simulink model "Non_linear_bicycle_model"  (R2020a)
settings: Solver=VariableStepAuto  StartTime=0.0  StopTime=10.0  RelTol=1e-3
values from neighbouring files (symbols this model uses):
  c_alpha_f = 156000    [init.m]
  c_alpha_r = 193000    [init.m]
  delta_max = deg2rad(37.3)    [init.m]
  g = 9.81    [init.m]
  Iz = 2937    [init.m]
  lf = 1.04    [init.m]
  lr = 1.40    (= 1.4)    [init.m]
  mass = 1919    [init.m]
  psi0 = 0*pi/180    (= 0)    [init.m]
  psid0 = 0    [init.m]
  steering_constant = deg2rad(10)    [init.m]
  steering_input_switch = 3    [init.m]
  steering_omega = 0.25    [init.m]
  steering_rate = deg2rad(2)    [init.m]
  v_lat0 = 0    [init.m]
  v_lon0 = 5    [init.m]
  wff = 0.577    [init.m]
  wfr = 0.423    [init.m]
  x0 = 0    [init.m]
  y0 = 0    [init.m]
undefined symbols (not defined in the file or in its folder): B_f, B_r, C_f, C_r, coefficient_friction, D_f, D_r, E_f, E_r
libraries: simulink x2
settings Model: Creator=Sameed Quais  LastModifiedBy=Sameed Quais

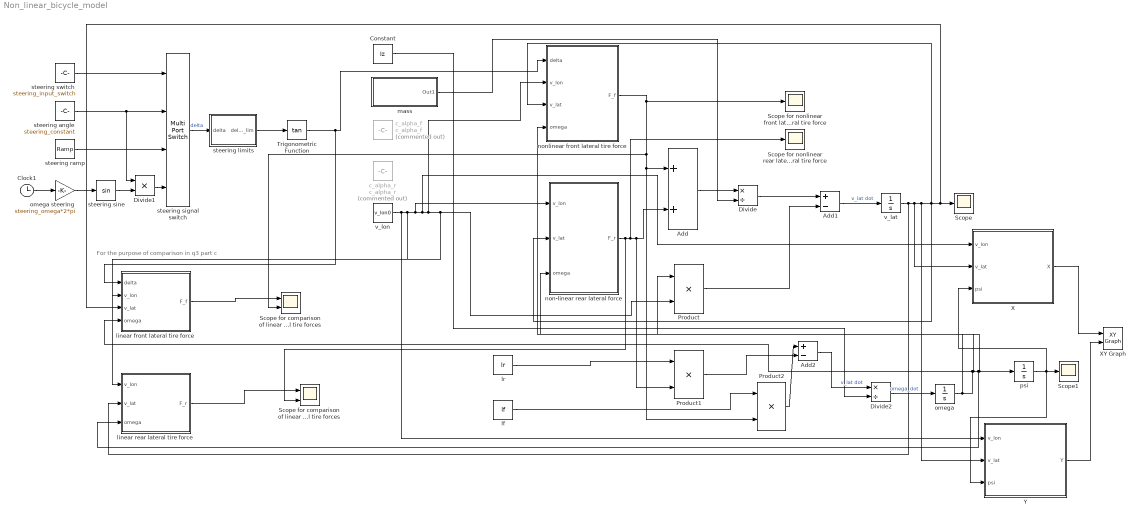
== system Non_linear_bicycle_model ==
  note: For the purpose of comparison in q3 part c
  Add : Sum
  Add1 : Sum  Inputs=+-
  Add2 : Sum  Inputs=+-
  Clock1 : Clock
  Constant : Constant  Value=Iz
  Divide : Product  Inputs=*/
  Divide1 : Product
  Divide2 : Product  Inputs=*/
  Product : Product
  Product1 : Product
  Product2 : Product
  Scope : Scope
  Scope for comparison of linear and non-linear front lateral tire forces : Scope  NumInputPorts=2
  Scope for comparison of linear and non-linear rear lateral tire forces : Scope  NumInputPorts=2
  Scope for nonlinear front lateral tire force : Scope
  Scope for nonlinear rear lateral tire force : Scope
  Scope1 : Scope
  Trigonometric Function : Trigonometry  Operator=tan
  X : Subsystem
  XY Graph : simulink/Sinks/XY Graph  xmin=-inf  xmax=inf  ymin=-inf  ymax=inf  st=-1
  Y : Subsystem
  c_alpha_f : Constant  Commented=on  Value=c_alpha_f
  c_alpha_r : Constant  Commented=on  Value=c_alpha_r
  lf : Constant  Value=lf
  linear front lateral tire force : Subsystem
  linear rear lateral tire force : Subsystem
  lr : Constant  Value=lr
  mass : Subsystem
  non-linear rear lateral force : Subsystem
  nonlinear front lateral tire force : Subsystem
  omega : Integrator  InitialCondition=psi0
  omega steering : Gain  Gain=steering_omega*2*pi
  psi : Integrator  InitialCondition=psid0
  steering angle : Constant  Value=steering_constant
  steering limits : Subsystem
  steering ramp : simulink/Sources/Ramp  slope=steering_rate  start=0  InitialOutput=0
  steering sine : Trigonometry
  steering switch : Constant  Value=steering_input_switch
  steering signal switch : MultiPortSwitch
  v_lat : Integrator  InitialCondition=v_lat0
  v_lon : Constant  Value=v_lon0
  wires:
  non-linear rear lateral force/1(F_r) -> Scope for nonlinear rear lateral tire force/1, Product1/2, Add/2, Scope for comparison of linear and non-linear rear lateral tire forces/2
  nonlinear front lateral tire force/1(F_f) -> Scope for comparison of linear and non-linear front lateral tire forces/2, Product2/2, Add/1, Scope for nonlinear front lateral tire force/1
  Add/1 -> Divide/1
  mass/1(Out1) -> Divide/2
  Divide/1 -> Add1/1
  v_lon/1 -> Y/1(v_lon), linear front lateral tire force/2(v_lon), non-linear rear lateral force/1(v_lon), X/1(v_lon), nonlinear front lateral tire force/2(v_lon), linear rear lateral tire force/1(v_lon), Product/2
  Product/1 -> Add1/2
  Add1/1 -> v_lat/1  "v_lat dot"
  lr/1 -> Product1/1
  lf/1 -> Product2/1
  Product2/1 -> Add2/1
  Product1/1 -> Add2/2
  Constant/1 -> Divide2/2
  Add2/1 -> Divide2/1  "v_lat dot"
  Divide2/1 -> omega/1  "omega_dot"
  v_lat/1 -> linear rear lateral tire force/2(v_lat), X/2(v_lat), Y/2(v_lat), non-linear rear lateral force/2(v_lat), nonlinear front lateral tire force/3(v_lat), linear front lateral tire force/3(v_lat), Scope/1
  omega/1 -> non-linear rear lateral force/3(omega), linear front lateral tire force/4(omega), Product/1, psi/1, nonlinear front lateral tire force/4(omega), linear rear lateral tire force/3(omega)
  steering limits/1(delta_lim) -> Trigonometric Function/1
  steering signal switch/1 -> steering limits/1(delta)  "delta"
  Clock1/1 -> omega steering/1
  steering angle/1 -> Divide1/1, steering signal switch/2
  Divide1/1 -> steering signal switch/4
  omega steering/1 -> steering sine/1
  steering switch/1 -> steering signal switch/1
  steering ramp/1 -> steering signal switch/3
  steering sine/1 -> Divide1/2
  Trigonometric Function/1 -> linear front lateral tire force/1(delta), nonlinear front lateral tire force/1(delta)
  psi/1 -> Y/3(psi), X/3(psi), Scope1/1
  X/1(X) -> XY Graph/1
  Y/1(Y) -> XY Graph/2
  linear front lateral tire force/1(F_f) -> Scope for comparison of linear and non-linear front lateral tire forces/1
  linear rear lateral tire force/1(F_r) -> Scope for comparison of linear and non-linear rear lateral tire forces/1

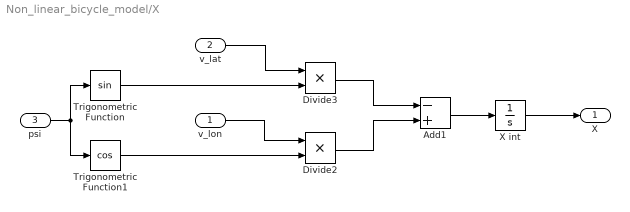
== system Non_linear_bicycle_model/X ==
  v_lon : Inport
  v_lat : Inport  Port=2
  psi : Inport  Port=3
  Add1 : Sum  Inputs=-+
  Divide2 : Product
  Divide3 : Product
  Trigonometric Function : Trigonometry
  Trigonometric Function1 : Trigonometry  Operator=cos
  X int : Integrator  InitialCondition=x0
  X : Outport  VectorParamsAs1DForOutWhenUnconnected=off
  wires:
  Add1/1 -> X int/1
  v_lon/1 -> Divide2/1
  Divide2/1 -> Add1/2
  v_lat/1 -> Divide3/1
  psi/1 -> Trigonometric Function/1, Trigonometric Function1/1
  Trigonometric Function1/1 -> Divide2/2
  Trigonometric Function/1 -> Divide3/2
  Divide3/1 -> Add1/1
  X int/1 -> X/1

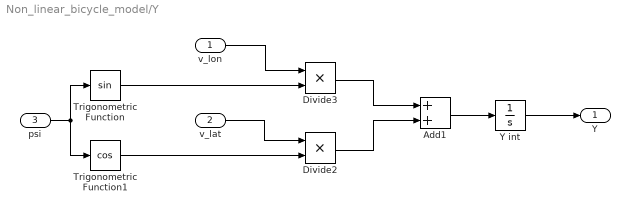
== system Non_linear_bicycle_model/Y ==
  v_lon : Inport
  v_lat : Inport  Port=2
  psi : Inport  Port=3
  Add1 : Sum
  Divide2 : Product
  Divide3 : Product
  Trigonometric Function : Trigonometry
  Trigonometric Function1 : Trigonometry  Operator=cos
  Y int : Integrator  InitialCondition=y0
  Y : Outport  VectorParamsAs1DForOutWhenUnconnected=off
  wires:
  Add1/1 -> Y int/1
  v_lat/1 -> Divide2/1
  Divide2/1 -> Add1/2
  v_lon/1 -> Divide3/1
  psi/1 -> Trigonometric Function/1, Trigonometric Function1/1
  Trigonometric Function1/1 -> Divide2/2
  Trigonometric Function/1 -> Divide3/2
  Divide3/1 -> Add1/1
  Y int/1 -> Y/1

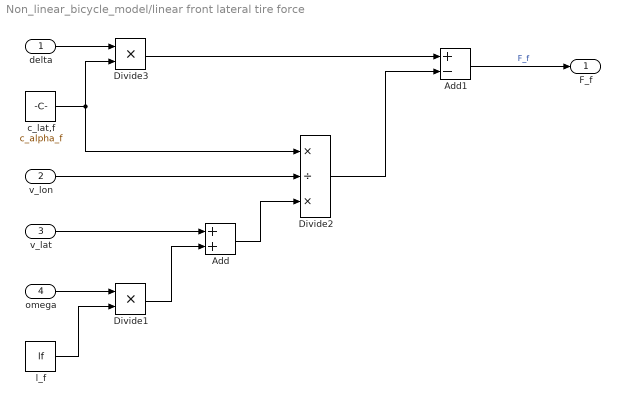
== system Non_linear_bicycle_model/linear front lateral tire force ==
  delta : Inport
  v_lon : Inport  Port=2
  v_lat : Inport  Port=3
  omega : Inport  Port=4
  Add : Sum
  Add1 : Sum  Inputs=+-
  Divide1 : Product
  Divide2 : Product  Inputs=*/*
  Divide3 : Product
  c_lat,f : Constant  Value=c_alpha_f
  l_f : Constant  Value=lf
  F_f : Outport  VectorParamsAs1DForOutWhenUnconnected=off
  wires:
  delta/1 -> Divide3/1
  c_lat,f/1 -> Divide2/1, Divide3/2
  omega/1 -> Divide1/1
  l_f/1 -> Divide1/2
  v_lat/1 -> Add/1
  Divide1/1 -> Add/2
  v_lon/1 -> Divide2/2
  Add/1 -> Divide2/3
  Divide2/1 -> Add1/2
  Divide3/1 -> Add1/1
  Add1/1 -> F_f/1  "F_f"

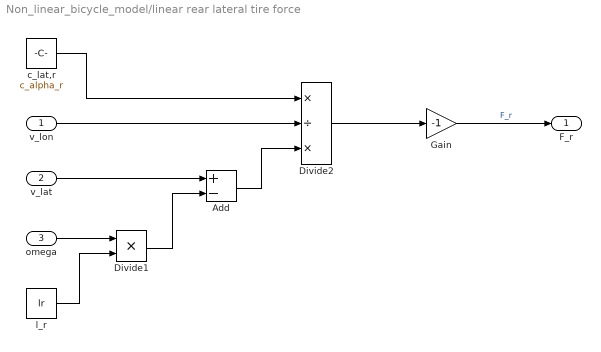
== system Non_linear_bicycle_model/linear rear lateral tire force ==
  v_lon : Inport
  v_lat : Inport  Port=2
  omega : Inport  Port=3
  Add : Sum  Inputs=+-
  Divide1 : Product
  Divide2 : Product  Inputs=*/*
  Gain : Gain  Gain=-1
  c_lat,r : Constant  Value=c_alpha_r
  l_r : Constant  Value=lr
  F_r : Outport  VectorParamsAs1DForOutWhenUnconnected=off
  wires:
  c_lat,r/1 -> Divide2/1
  omega/1 -> Divide1/1
  l_r/1 -> Divide1/2
  v_lat/1 -> Add/1
  Divide1/1 -> Add/2
  v_lon/1 -> Divide2/2
  Add/1 -> Divide2/3
  Divide2/1 -> Gain/1
  Gain/1 -> F_r/1  "F_r"

== system Non_linear_bicycle_model/mass ==
  mass : Constant  Value=mass
  Out1 : Outport
  wires:
  mass/1 -> Out1/1

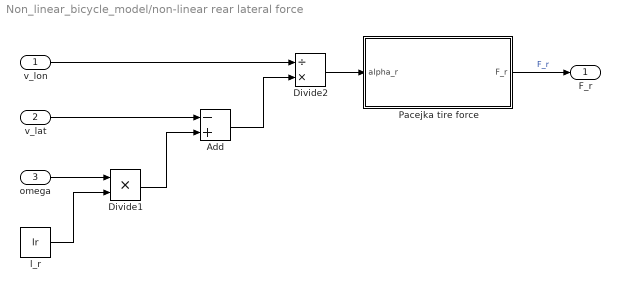
== system Non_linear_bicycle_model/non-linear rear lateral force ==
  v_lon : Inport
  v_lat : Inport  Port=2
  omega : Inport  Port=3
  Add : Sum  Inputs=-+
  Divide1 : Product
  Divide2 : Product  Inputs=/*
  Pacejka tire force : Subsystem
  l_r : Constant  Value=lr
  F_r : Outport  VectorParamsAs1DForOutWhenUnconnected=off
  wires:
  v_lon/1 -> Divide2/1
  Pacejka tire force/1(F_r) -> F_r/1  "F_r"
  l_r/1 -> Divide1/2
  Divide1/1 -> Add/2
  Divide2/1 -> Pacejka tire force/1(alpha_r)
  Add/1 -> Divide2/2
  v_lat/1 -> Add/1
  omega/1 -> Divide1/1

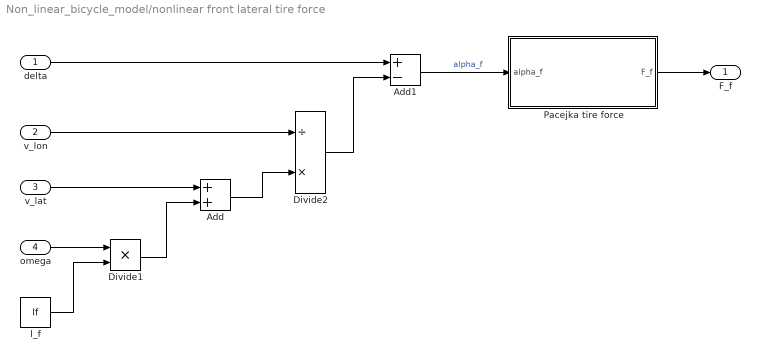
== system Non_linear_bicycle_model/nonlinear front lateral tire force ==
  delta : Inport
  v_lon : Inport  Port=2
  v_lat : Inport  Port=3
  omega : Inport  Port=4
  Add : Sum
  Add1 : Sum  Inputs=+-
  Divide1 : Product
  Divide2 : Product  Inputs=/*
  Pacejka tire force : Subsystem
  l_f : Constant  Value=lf
  F_f : Outport
  wires:
  Divide1/1 -> Add/2
  Divide2/1 -> Add1/2
  omega/1 -> Divide1/1
  l_f/1 -> Divide1/2
  Add/1 -> Divide2/2
  v_lon/1 -> Divide2/1
  v_lat/1 -> Add/1
  delta/1 -> Add1/1
  Add1/1 -> Pacejka tire force/1(alpha_f)  "alpha_f"
  Pacejka tire force/1(F_f) -> F_f/1

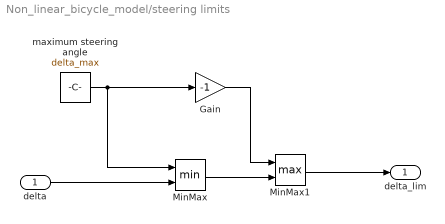
== system Non_linear_bicycle_model/steering limits ==
  delta : Inport
  Gain : Gain  Gain=-1
  MinMax : MinMax  Inputs=2
  MinMax1 : MinMax  Function=max  Inputs=2
  maximum steering angle : Constant  Value=delta_max
  delta_lim : Outport  VectorParamsAs1DForOutWhenUnconnected=off
  wires:
  MinMax1/1 -> delta_lim/1
  delta/1 -> MinMax/2
  maximum steering angle/1 -> Gain/1, MinMax/1
  MinMax/1 -> MinMax1/2
  Gain/1 -> MinMax1/1

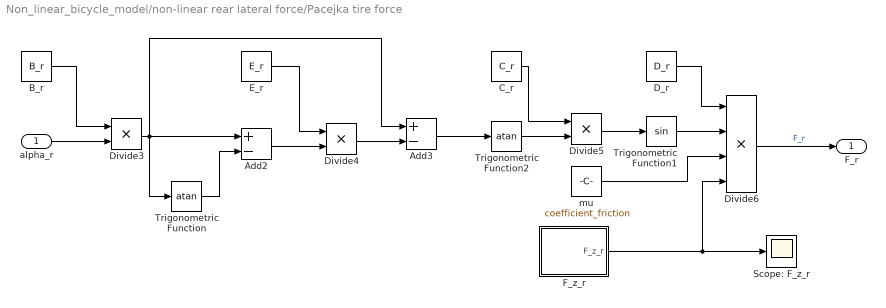
== system Non_linear_bicycle_model/non-linear rear lateral force/Pacejka tire force ==
  alpha_r : Inport
  Add2 : Sum  Inputs=+-
  Add3 : Sum  Inputs=+-
  B_r : Constant  Value=B_r
  C_r : Constant  Value=C_r
  D_r : Constant  Value=D_r
  Divide3 : Product
  Divide4 : Product
  Divide5 : Product
  Divide6 : Product  Inputs=4
  E_r : Constant  Value=E_r
  F_z_r : Subsystem
  Scope: F_z_r : Scope
  Trigonometric Function : Trigonometry  Operator=atan
  Trigonometric Function1 : Trigonometry
  Trigonometric Function2 : Trigonometry  Operator=atan
  mu : Constant  Value=coefficient_friction
  F_r : Outport  VectorParamsAs1DForOutWhenUnconnected=off
  wires:
  Divide6/1 -> F_r/1  "F_r"
  Divide3/1 -> Add2/1, Add3/1, Trigonometric Function/1
  Divide4/1 -> Add3/2
  Trigonometric Function1/1 -> Divide6/2
  Trigonometric Function/1 -> Add2/2
  Divide5/1 -> Trigonometric Function1/1
  C_r/1 -> Divide5/1
  mu/1 -> Divide6/3
  Add3/1 -> Trigonometric Function2/1
  D_r/1 -> Divide6/1
  B_r/1 -> Divide3/1
  E_r/1 -> Divide4/1
  alpha_r/1 -> Divide3/2
  Add2/1 -> Divide4/2
  F_z_r/1(F_z_r) -> Divide6/4, Scope: F_z_r/1
  Trigonometric Function2/1 -> Divide5/2

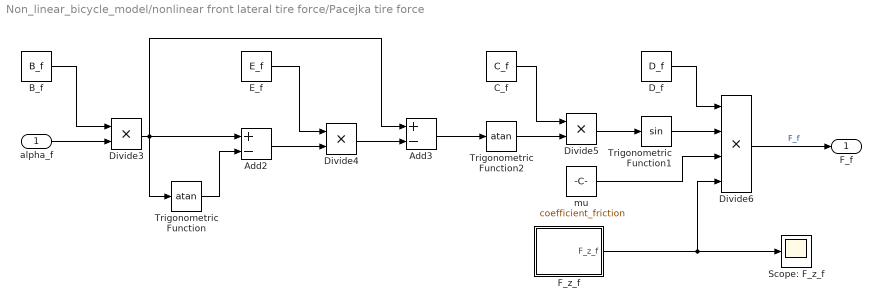
== system Non_linear_bicycle_model/nonlinear front lateral tire force/Pacejka tire force ==
  alpha_f : Inport
  Add2 : Sum  Inputs=+-
  Add3 : Sum  Inputs=+-
  B_f : Constant  Value=B_f
  C_f : Constant  Value=C_f
  D_f : Constant  Value=D_f
  Divide3 : Product
  Divide4 : Product
  Divide5 : Product
  Divide6 : Product  Inputs=4
  E_f : Constant  Value=E_f
  F_z_f : Subsystem
  Scope: F_z_f : Scope
  Trigonometric Function : Trigonometry  Operator=atan
  Trigonometric Function1 : Trigonometry
  Trigonometric Function2 : Trigonometry  Operator=atan
  mu : Constant  Value=coefficient_friction
  F_f : Outport  VectorParamsAs1DForOutWhenUnconnected=off
  wires:
  Divide6/1 -> F_f/1  "F_f"
  Divide3/1 -> Add2/1, Add3/1, Trigonometric Function/1
  Divide4/1 -> Add3/2
  Trigonometric Function1/1 -> Divide6/2
  Trigonometric Function/1 -> Add2/2
  Divide5/1 -> Trigonometric Function1/1
  C_f/1 -> Divide5/1
  mu/1 -> Divide6/3
  Add3/1 -> Trigonometric Function2/1
  D_f/1 -> Divide6/1
  B_f/1 -> Divide3/1
  E_f/1 -> Divide4/1
  alpha_f/1 -> Divide3/2
  Add2/1 -> Divide4/2
  F_z_f/1(F_z_f) -> Scope: F_z_f/1, Divide6/4
  Trigonometric Function2/1 -> Divide5/2

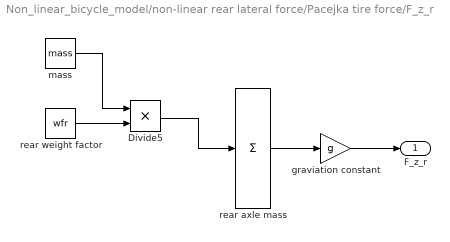
== system Non_linear_bicycle_model/non-linear rear lateral force/Pacejka tire force/F_z_r ==
  Divide5 : Product
  graviation constant : Gain  Gain=g
  mass : Constant  Value=mass
  rear axle mass : Sum  Inputs=+
  rear weight factor : Constant  Value=wfr
  F_z_r : Outport  VectorParamsAs1DForOutWhenUnconnected=off
  wires:
  rear axle mass/1 -> graviation constant/1
  mass/1 -> Divide5/1
  rear weight factor/1 -> Divide5/2
  Divide5/1 -> rear axle mass/1
  graviation constant/1 -> F_z_r/1

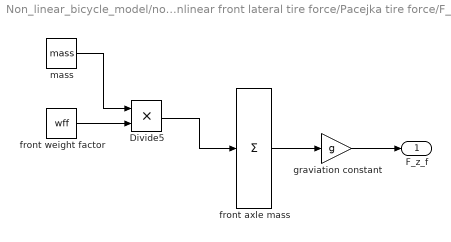
== system Non_linear_bicycle_model/nonlinear front lateral tire force/Pacejka tire force/F_z_f ==
  Divide5 : Product
  front axle mass : Sum  Inputs=+
  front weight factor : Constant  Value=wff
  graviation constant : Gain  Gain=g
  mass : Constant  Value=mass
  F_z_f : Outport  VectorParamsAs1DForOutWhenUnconnected=off
  wires:
  front axle mass/1 -> graviation constant/1
  mass/1 -> Divide5/1
  front weight factor/1 -> Divide5/2
  Divide5/1 -> front axle mass/1
  graviation constant/1 -> F_z_f/1
